simulink model "poroject_matlab1"  (R2021a)
settings: Solver=FixedStepAuto  StartTime=0.0  StopTime=T  FixedStep=0.1  RelTol=1e-3
values from neighbouring files (symbols this model uses):
  C1 = 1    [untitled.m]
  C2 = 1    [untitled.m]
  R1 = 1    [untitled.m]
  R2 = 1    [untitled.m]
  x = 1    [untitled.m]
undefined symbols (not defined in the file or in its folder): Amplitude, W
libraries: simulink_extras x9, spsSeriesRLCBranchLib x4, simulink x2, spsCurrentMeasurementLib x1, spsDCVoltageSourceLib x1, spsVoltageMeasurementLib x1, spspowerguiLib x1
settings Model: Creator=sh  LastModifiedBy=solo

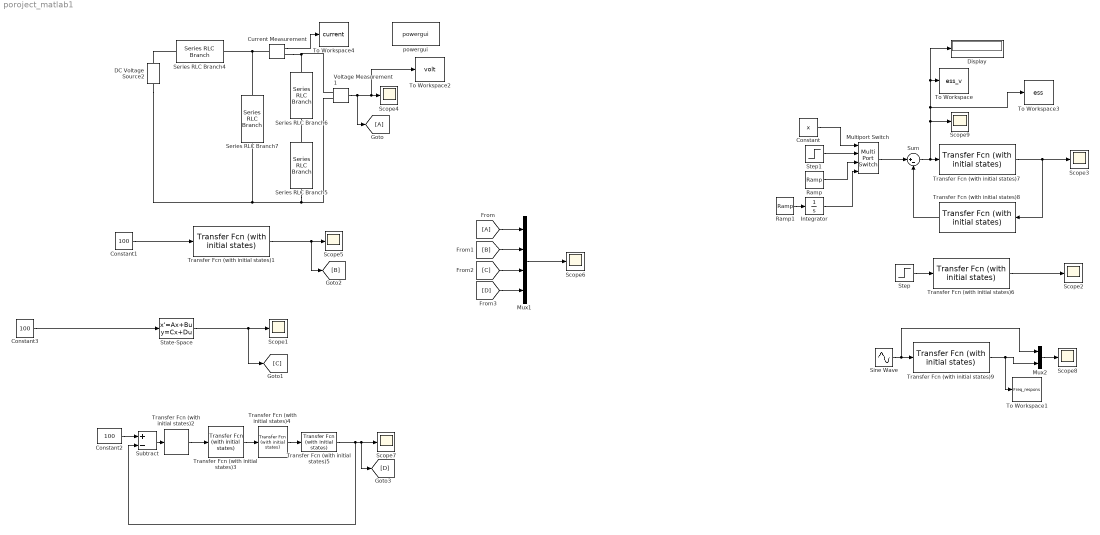
== system poroject_matlab1 ==
  Constant : Constant  Value=x
  Constant1 : Constant  Value=100
  Constant2 : Constant  Value=100
  Constant3 : Constant  Value=100
  Current Measurement : spsCurrentMeasurementLib/Current Measurement  PhasorSimulation=off  OutputType=Complex  PSBequivalent=0
  DC Voltage Source2 : spsDCVoltageSourceLib/DC Voltage Source  Amplitude=100  Measurements=None
  Display : Display
  Integrator : Integrator
  Multiport Switch : MultiPortSwitch
  Mux1 : Mux
  Mux2 : Mux  Inputs=2
  Ramp : simulink/Sources/Ramp  slope=1  start=0  InitialOutput=0
  Ramp1 : simulink/Sources/Ramp  slope=1  start=0  InitialOutput=0
  Scope{1..9} (9 alike) : Scope
  Series RLC Branch4 : spsSeriesRLCBranchLib/Series RLC Branch  LConnTagsString=__new0  RConnTagsString=__new0  BranchType=R  Resistance=R1  Inductance=1e-3  SetiL0=off  InitialCurrent=0  Capacitance=1e-6  Setx0=off  InitialVoltage=0  Measurements=None
  Series RLC Branch5 : spsSeriesRLCBranchLib/Series RLC Branch  LConnTagsString=__new0  RConnTagsString=__new0  BranchType=C  Resistance=4  Inductance=1e-3  SetiL0=off  InitialCurrent=0  Capacitance=C2  Setx0=on  InitialVoltage=0  Measurements=None
  Series RLC Branch6 : spsSeriesRLCBranchLib/Series RLC Branch  LConnTagsString=__new0  RConnTagsString=__new0  BranchType=R  Resistance=R2  Inductance=1e-3  SetiL0=off  InitialCurrent=0  Capacitance=1e-6  Setx0=off  InitialVoltage=0  Measurements=None
  Series RLC Branch7 : spsSeriesRLCBranchLib/Series RLC Branch  LConnTagsString=__new0  RConnTagsString=__new0  BranchType=C  Resistance=4  Inductance=1e-3  SetiL0=off  InitialCurrent=0  Capacitance=C1  Setx0=on  InitialVoltage=0  Measurements=None
  Sine Wave : Sin  Amplitude=Amplitude  Frequency=W  SampleTime=0
  State-Space : StateSpace  A="[0  1 ;-1/90  -29/90]"  B="[0  ; 1/90]"  C="[1  18]"  D=0  InitialCondition=0
  Step : Step  Time=0  SampleTime=0
  Step1 : Step  Time=0  SampleTime=0
  Subtract : Sum  Inputs=+-
  Sum : Sum  Inputs=|+-
  To Workspace : ToWorkspace  VariableName=ess_v  SaveFormat=Structure  SampleTime=-1
      settings: Save2DSignal=2-D array (concatenate along first dimension)
  To Workspace1 : ToWorkspace  VariableName=Freq_respons  SaveFormat=Timeseries  SampleTime=-1
      settings: Save2DSignal=2-D array (concatenate along first dimension)
  To Workspace2 : ToWorkspace  VariableName=volt  SaveFormat=Timeseries  SampleTime=-1
      settings: Save2DSignal=2-D array (concatenate along first dimension)
  To Workspace3 : ToWorkspace  VariableName=ess  SaveFormat=Timeseries  SampleTime=-1
      settings: Save2DSignal=2-D array (concatenate along first dimension)
  To Workspace4 : ToWorkspace  VariableName=current  SaveFormat=Timeseries  SampleTime=-1
      settings: Save2DSignal=2-D array (concatenate along first dimension)
  Transfer Fcn (with initial states)1 : simulink_extras/Additional Linear/Transfer Fcn (with initial states)  N=[18 1]  D=[90 29 1]  X0=0
  Transfer Fcn (with initial states)2 : simulink_extras/Additional Linear/Transfer Fcn (with initial states)  N=[1]  D=[ 1]  X0=0
  Transfer Fcn (with initial states)3 : simulink_extras/Additional Linear/Transfer Fcn (with initial states)  N=[1]  D=[ 5 0]  X0=0
  Transfer Fcn (with initial states)4 : simulink_extras/Additional Linear/Transfer Fcn (with initial states)  N=[18 1]  D=[6 0]  X0=0
  Transfer Fcn (with initial states)5 : simulink_extras/Additional Linear/Transfer Fcn (with initial states)  N=[30 0 0]  D=[90 11 0]  X0=0
  Transfer Fcn (with initial states)6 : simulink_extras/Additional Linear/Transfer Fcn (with initial states)  N=[0.155]  D=[1 0.37 0.155]  X0=0
  Transfer Fcn (with initial states)7 : simulink_extras/Additional Linear/Transfer Fcn (with initial states)  N="[ (C2*R2)    1]"  D="[ (R1*R2*C1*C2 )    (R1*C2+R1*C1)      0]"  X0=0
  Transfer Fcn (with initial states)8 : simulink_extras/Additional Linear/Transfer Fcn (with initial states)  N=[1]  D=[1]  X0=0
  Transfer Fcn (with initial states)9 : simulink_extras/Additional Linear/Transfer Fcn (with initial states)  N=[18 1]  D=[90 29 1]  X0=0
  Voltage Measurement1 : spsVoltageMeasurementLib/Voltage Measurement  PhasorSimulation=off  OutputType=Complex  PSBequivalent=0
  powergui : spspowerguiLib/powergui  Priority=1  SimulationMode=Continuous  SampleTime=50e-6  frequency=60  Iterations=50  frequencyindice=0  Pbase=100e6  ErrMax=1e-4  UnitsV=kV  UnitsW=MW  buscounter=0  FunctionMessages=off  echomessages=off  EnableUseOfTLC=off  CurrentSourceSwitches=off  DisableSnubberDevices=off  DisableRonSwitches=off  DisableVfSwitches=off  DisplayEquations=off  AutomaticDiscreteSolvers=off  SolverType=Tustin/Backward Euler (TBE)  Interpol=off  ExternalGateDelay=off  methode=off  Ts=100  x0status=blocks  SPID=on  SwTol=0  HookPort=off  NonlinearTolerance=1e-4  nMaxIteration=100  ContinueOnMaxIteration=off  RestoreLinks=warning  ResistiveCurrentMeasurement=off  Frange=[0:2:500]  Ylog=off  Xlog=on  ShowGrid=off  save=off  variable=ZData  structure=0  ZoomFFT=off  StartTime=0.0  cycles=1  DisplayStyle=1  fundamental=60  FreqAxis=off  MaxFrequency=1000  frequencyindicesteady=1  RmsSteady=1  display=off
  wires:
  Voltage Measurement1/1 -> [A], To Workspace2/1, Scope4/1
  Constant1/1 -> Transfer Fcn (with initial states)1/1
  Transfer Fcn (with initial states)1/1 -> [B], Scope5/1
  Mux1/1 -> Scope6/1
  Transfer Fcn (with initial states)2/1 -> Transfer Fcn (with initial states)3/1
  Transfer Fcn (with initial states)3/1 -> Transfer Fcn (with initial states)4/1
  Transfer Fcn (with initial states)4/1 -> Transfer Fcn (with initial states)5/1
  Subtract/1 -> Transfer Fcn (with initial states)2/1
  Transfer Fcn (with initial states)5/1 -> Subtract/2, [D], Scope7/1
  Constant3/1 -> State-Space/1
  State-Space/1 -> [C], Scope1/1
  Transfer Fcn (with initial states)6/1 -> Scope2/1
  Step/1 -> Transfer Fcn (with initial states)6/1
  Transfer Fcn (with initial states)7/1 -> Transfer Fcn (with initial states)8/1, Scope3/1
  Sum/1 -> Scope9/1, Display/1, To Workspace/1, To Workspace3/1, Transfer Fcn (with initial states)7/1
  Transfer Fcn (with initial states)8/1 -> Sum/2
  Constant2/1 -> Subtract/1
  Mux2/1 -> Scope8/1
  Transfer Fcn (with initial states)9/1 -> To Workspace1/1, Mux2/2
  Sine Wave/1 -> Mux2/1, Transfer Fcn (with initial states)9/1
  [A] -> Mux1/1
  [B] -> Mux1/2
  [C] -> Mux1/3
  [D] -> Mux1/4
  Current Measurement/1 -> To Workspace4/1
  Multiport Switch/1 -> Sum/1
  Step1/1 -> Multiport Switch/2
  Ramp/1 -> Multiport Switch/3
  Ramp1/1 -> Integrator/1
  Integrator/1 -> Multiport Switch/4
  Constant/1 -> Multiport Switch/1
  connections:
  DC Voltage Source2/RConn1 -- Series RLC Branch4/LConn1
  Series RLC Branch5/LConn1 -- Series RLC Branch6/RConn1
  Voltage Measurement1/LConn1 -- Current Measurement/RConn1 -- Series RLC Branch6/LConn1
  Series RLC Branch5/RConn1 -- Voltage Measurement1/LConn2 -- DC Voltage Source2/LConn1 -- Series RLC Branch7/RConn1
  Series RLC Branch7/LConn1 -- Current Measurement/LConn1 -- Series RLC Branch4/RConn1
